simulink model "Control_System"  (R2025b)
settings: Solver=VariableStepDiscrete  StartTime=0.0  StopTime=10.0  RelTol=1e-3
settings Model: Creator=samue  LastModifiedBy=samue

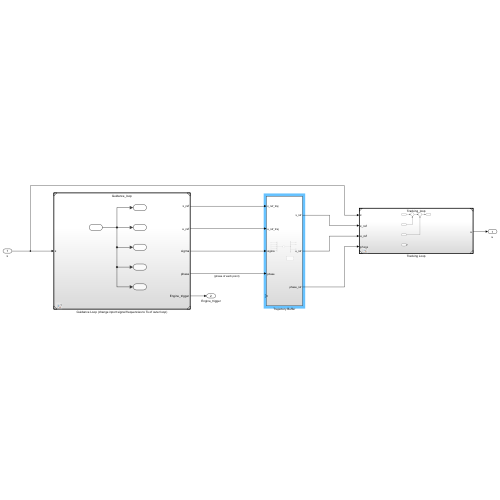
[thumbnail: Simulink's stored preview of the top-level diagram]
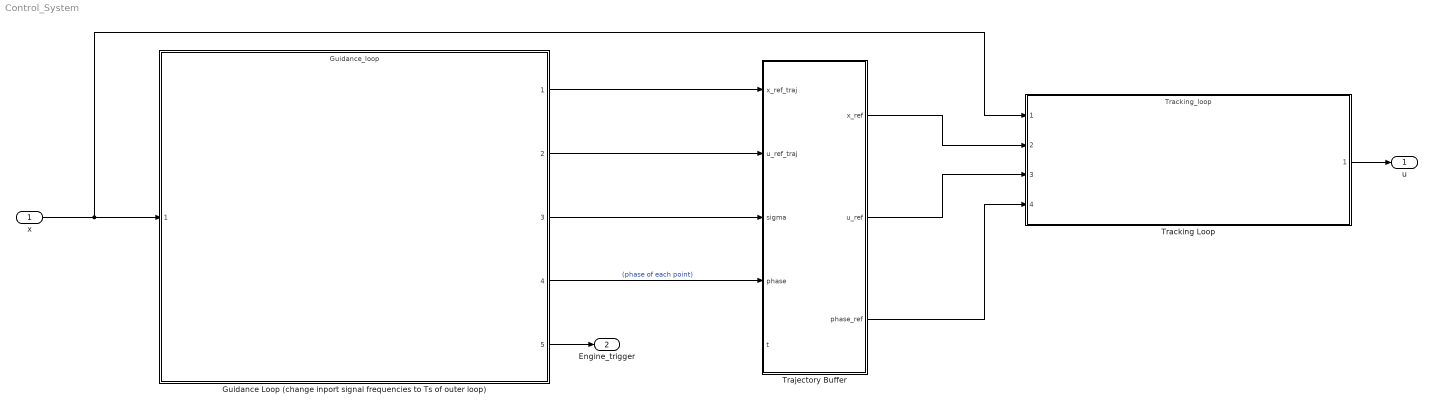
== system Control_System ==
  x : Inport
  Guidance Loop (change inport signal frequencies to Ts of outer loop) : ModelReference  ModelNameDialog=Guidance_loop.slx  SimulationMode=Normal  ModelReferenceVersion=1.3
  Tracking Loop : ModelReference  ModelNameDialog=Tracking_loop.slx  SimulationMode=Normal  ModelReferenceVersion=1.6
  Trajectory Buffer : Subsystem
  u : Outport
  Engine_trigger : Outport  Port=2
  wires:
  x/1 -> Tracking Loop/1, Guidance Loop (change inport signal frequencies to Ts of outer loop)/1
  Guidance Loop (change inport signal frequencies to Ts of outer loop)/5 -> Engine_trigger/1
  Guidance Loop (change inport signal frequencies to Ts of outer loop)/1 -> Trajectory Buffer/1(x_ref_traj)
  Guidance Loop (change inport signal frequencies to Ts of outer loop)/2 -> Trajectory Buffer/2(u_ref_traj)
  Guidance Loop (change inport signal frequencies to Ts of outer loop)/3 -> Trajectory Buffer/3(sigma)
  Guidance Loop (change inport signal frequencies to Ts of outer loop)/4 -> Trajectory Buffer/4(phase)  "(phase of each point)"
  Tracking Loop/1 -> u/1
  Trajectory Buffer/1(x_ref) -> Tracking Loop/2
  Trajectory Buffer/2(u_ref) -> Tracking Loop/3
  Trajectory Buffer/3(phase_ref) -> Tracking Loop/4

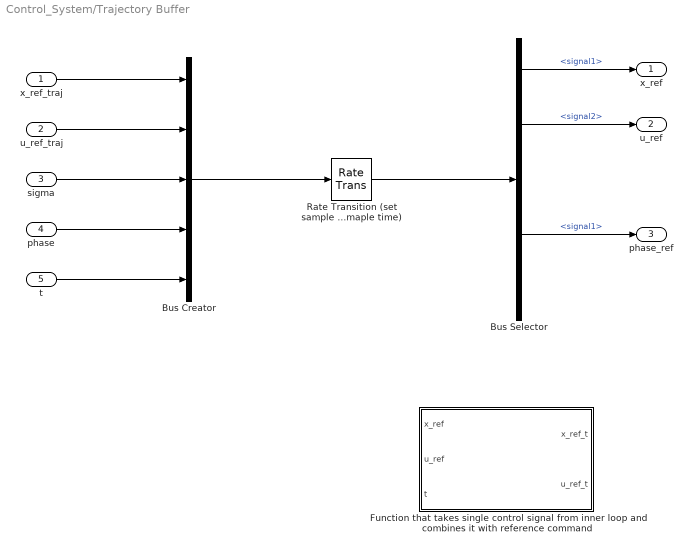
== system Control_System/Trajectory Buffer ==
  x_ref_traj : Inport
  u_ref_traj : Inport  Port=2
  sigma : Inport  Port=3
  phase : Inport  Port=4
  t : Inport  Port=5
  Bus Creator : BusCreator  Inputs=5
  Bus Selector : BusSelector  OutputSignals=signal1,signal2,signal3,signal1,signal2
  Function that takes single control signal from inner loop and combines it with reference command : MATLAB Function  TreatAsAtomicUnit=on
  Rate Transition (set sample time to inner loop smaple time) : RateTransition
  x_ref : Outport
  u_ref : Outport  Port=2
  phase_ref : Outport  Port=3
  wires:
  x_ref_traj/1 -> Bus Creator/1
  u_ref_traj/1 -> Bus Creator/2
  sigma/1 -> Bus Creator/3
  phase/1 -> Bus Creator/4
  t/1 -> Bus Creator/5
  Bus Creator/1 -> Rate Transition (set sample time to inner loop smaple time)/1
  Rate Transition (set sample time to inner loop smaple time)/1 -> Bus Selector/1
  Bus Selector/2 -> u_ref/1  "<signal2>"
  Bus Selector/1 -> x_ref/1  "<signal1>"
  Bus Selector/4 -> phase_ref/1  "<signal1>"

== matlab function Control_System/Trajectory Buffer/Function that takes single control signal from inner loop and combines it with reference command ==
  data: x_ref input; u_ref input; x_ref_t output; u_ref_t output; t input
function [x_ref_t, u_ref_t] = target_selector(x_ref, u_ref, t)
% Take full trajectory and current time and extracts relevent reference
end
